simulink model "SIM_nominal"  (R2023b)
settings: Solver=VariableStepAuto  StartTime=0.0  StopTime=500  RelTol=1e-3
values from neighbouring files (symbols this model uses):
  Ts = 0.1    [NMPC_conFer.m]
libraries: mpclib x1
settings Model: Creator=akeebismail  LastModifiedBy=akeebismail

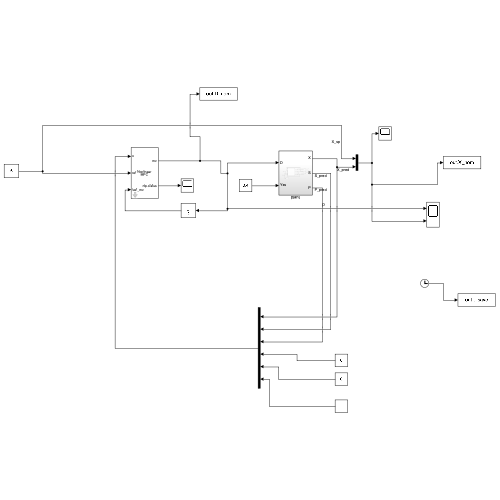
[thumbnail: Simulink's stored preview of the top-level diagram]
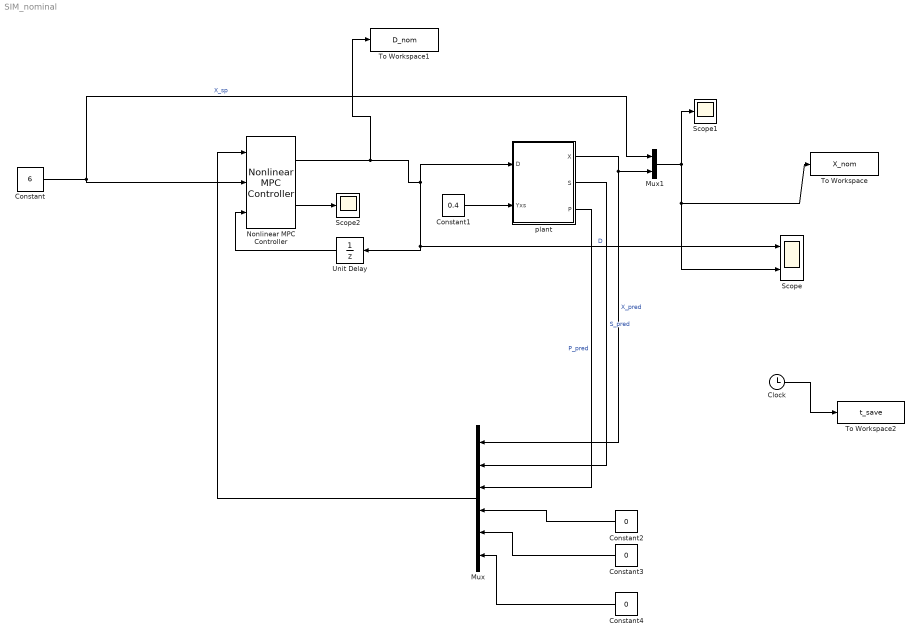
== system SIM_nominal ==
  Clock : Clock
  Constant : Constant  Value=6
  Constant1 : Constant  Value=0.4
  Constant2 : Constant  Value=0
  Constant3 : Constant  Value=0
  Constant4 : Constant  Value=0
  Mux : Mux  Inputs=6
  Mux1 : Mux  Inputs=2
  Nonlinear MPC Controller : mpclib/Nonlinear MPC Controller  nlmpcobj=nlobj  UseObjectTs=on  UseMEX=off  md_enabled=off  mvtarget_enabled=off  param_enabled=off  cost_enabled=off  mvseq_enabled=off  stateseq_enabled=off  ovseq_enabled=off  slack_enabled=off  status_enabled=on  ov_min=off  ov_max=off  mv_min=off  mv_max=off  mvrate_min=off  mvrate_max=off  state_min=off  state_max=off  ov_weight=off  mv_weight=off  mvrate_weight=off  ecr_weight=off  nlp_initialize=off
  Scope : Scope  NumInputPorts=2
  Scope1 : Scope
  Scope2 : Scope
  To Workspace : ToWorkspace  VariableName=X_nom  SaveFormat=Timeseries  SampleTime=Ts
  To Workspace1 : ToWorkspace  VariableName=D_nom  SaveFormat=Timeseries  SampleTime=Ts
  To Workspace2 : ToWorkspace  VariableName=t_save  SaveFormat=Timeseries  SampleTime=Ts
  Unit Delay : UnitDelay  InitialCondition=0.202  SampleTime=Ts  HasFrameUpgradeWarning=on
  plant : Subsystem
  wires:
  plant/3(P) -> Mux/3  "P_pred"
  plant/2(S) -> Mux/2  "S_pred"
  Mux/1 -> Nonlinear MPC Controller/1
  Nonlinear MPC Controller/2 -> Scope2/1
  Constant/1 -> Nonlinear MPC Controller/2, Mux1/1  "X_sp"
  plant/1(X) -> Mux/1, Mux1/2  "X_pred"
  Nonlinear MPC Controller/1 -> To Workspace1/1, Scope/1, Unit Delay/1, plant/1(D)  "D"
  Mux1/1 -> Scope/2, To Workspace/1, Scope1/1
  Unit Delay/1 -> Nonlinear MPC Controller/3
  Constant1/1 -> plant/2(Yxs)
  Constant2/1 -> Mux/4
  Constant3/1 -> Mux/5
  Constant4/1 -> Mux/6
  Clock/1 -> To Workspace2/1

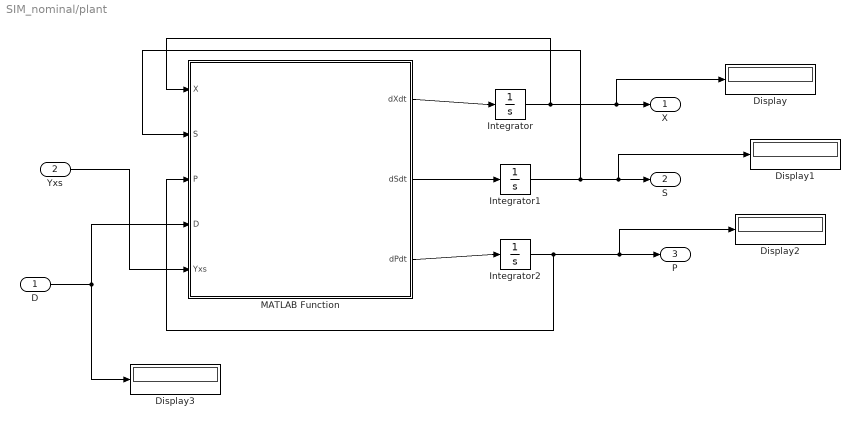
== system SIM_nominal/plant ==
  D : Inport
  Yxs : Inport  Port=2
  Display{,1..3} (4 alike) : Display
  Integrator : Integrator  InitialCondition=5
  Integrator1 : Integrator  InitialCondition=5
  Integrator2 : Integrator  InitialCondition=19.14
  MATLAB Function : MATLAB Function  TreatAsAtomicUnit=on
  X : Outport
  S : Outport  Port=2
  P : Outport  Port=3
  wires:
  MATLAB Function/1(dXdt) -> Integrator/1
  MATLAB Function/3(dPdt) -> Integrator2/1
  MATLAB Function/2(dSdt) -> Integrator1/1
  D/1 -> Display3/1, MATLAB Function/4(D)
  Integrator/1 -> Display/1, X/1, MATLAB Function/1(X)
  Integrator2/1 -> Display2/1, P/1, MATLAB Function/3(P)
  Integrator1/1 -> Display1/1, S/1, MATLAB Function/2(S)
  Yxs/1 -> MATLAB Function/5(Yxs)

== matlab function SIM_nominal/plant/MATLAB Function ==
  data: X input; dXdt output; S input; P input; D input; dSdt output; dPdt output; Yxs input
function [dXdt,dSdt,dPdt] = continuous_fermenter(X,S,P,D,Yxs)

values = {22,1.2,50,20,2.2,0.2,0.48};

[Ki,Km,Pm,Sf,alpha,beta,miu_m] = values{:};


miu = (miu_m * (1 - (P/Pm))) * S / (Km + S + (S^2 / Ki))  ;

dXdt = -D * X + miu * X     ;

dSdt = D * (Sf - S) - (1/Yxs) * miu * X   ;

dPdt = -D * P + (alpha * miu + beta) * X   ;

end
